simulink model "Fig434"  (R2014b)
settings: Solver=FixedStepDiscrete  StartTime=0.0  StopTime=0.524288  FixedStep=1e-6  RelTol=1e-3
libraries: commanapbnd3 x1
settings Model: DataTypeOverride=Double  MinMaxOverflowLogging=ForceOff  Creator=Dennis Silage  LastModifiedBy=Silage
settings DataIOCC: SignalLoggingSaveFormat=ModelDataLogs
settings OptimizationCC: ExpressionDepthLimit=2147483647  InitFltsAndDblsToZero=on
settings DebuggingCC: UnderspecifiedInitializationDetection=Classic  MergeDetectMultiDrivingBlocksExec=none  SolverPrmCheckMsg=none  FcnCallInpInsideContextMsg=UseLocalSettings  UnconnectedOutputMsg=none  StateNameClashWarn=warning
settings GRTTargetCC: CombineOutputUpdateFcns=off  GRTInterface=on

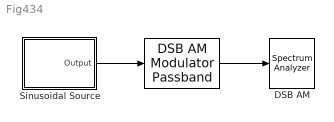
== system Fig434 ==
  "  " : commanapbnd3/DSB AM Modulator Passband  Fc=20000  Ph=-pi/2  Offset=1.5
  DSB AM : SpectrumAnalyzer
  Sinusoidal Source : Subsystem
  wires:
  Sinusoidal Source/1(Output) -> "  "/1
  "  "/1 -> DSB AM/1

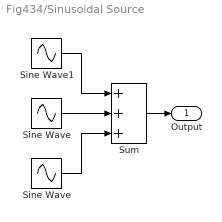
== system Fig434/Sinusoidal Source ==
  " Sine Wave " : Sin  Amplitude=0.2  Frequency=5000*pi  SampleTime=1e-6
  "Sine Wave " : Sin  Amplitude=0.5  Frequency=3000*pi  SampleTime=1e-6
  Sine Wave1 : Sin  Frequency=1000*pi  SampleTime=1e-6
  Sum : Sum  Inputs=+++
  Output : Outport
  wires:
  "Sine Wave "/1 -> Sum/2
  " Sine Wave "/1 -> Sum/3
  Sine Wave1/1 -> Sum/1
  Sum/1 -> Output/1
